simulink model "TestComputeProfileSource"  (R2025b)
settings: Solver=ode23t  StartTime=0.0  StopTime=15  MaxStep=1e-3  RelTol=1e-4
libraries: nesl_utility x5, fl_lib x1, datacenter_lib x1, simulink x1
settings Model: Creator=saprasad  LastModifiedBy=saprasad
settings SimscapeCC: SimscapeLogType=all  SimscapeLogName=simlog_TestComputeProfileSource  SimscapeLogLimitData=off

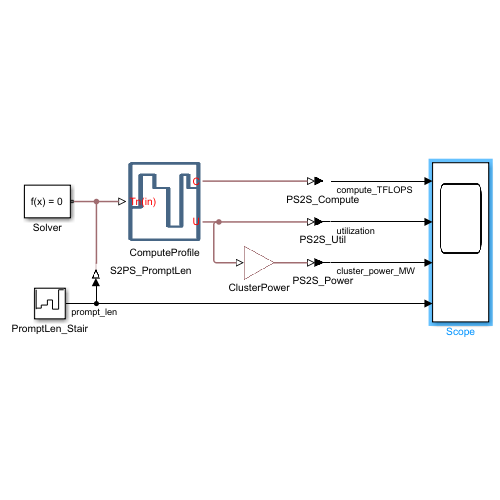
[thumbnail: Simulink's stored preview of the top-level diagram]
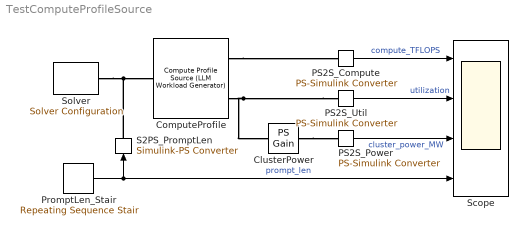
== system TestComputeProfileSource ==
  ClusterPower : fl_lib/Physical Signals/Functions/PS Gain  gain=1000 J/s
  ComputeProfile : datacenter_lib/Compute Profile Source (LLM Workload Generator)  gpuModel=GPUModel.B200  numGPUs=5184  workloadType=WorkloadType.Training  timeScale=10  tokenSource=TokenSource.External  showAdvanced=true  customPeakTFLOPS=1000  customHbmBW=4e12 1/s  hbmBW=8e12 1/s  interNodeBW=50e9 1/s  llmSize=LLMModelSize.GPT_175B  customNumParams_B=70  customNumLayers=80  customPrecision=2  parallelism=ParallelismStrategy.TP8_PP4  customTP=8  customPP=4  microBatch=8  globalBatch=12288  seqLength=2048  idleUtil=0.60  fwdUtil=0.92  bwdUtil=0.98  commSyncUtil=0.65  prompt_tokens=512  output_tokens=256  num_concurrent=8  batch_size=8  allreduce_latency=5e-6 s  baseInfUtil=0.08  baseInfFrac=0.10  MFU=0.85  checkpointOverhead=0.03  stragglerOverhead=0.02  trainableParamFrac=0.02  evalInterval=5  evalBatches=2  ft_checkpointOverhead=0.05  enableNoise=true  noiseAmplitude=0.05  stepJitter=0  enableFilter=false  filterTimeConstant=0.01 s  t_step_specify=off  t_step_priority=Low  t_step=0 s  t_step_nominal_specify=off  t_step_nominal_value=1  t_step_nominal_unit=s  phase_id_specify=off  phase_id_priority=None  phase_id=0  phase_id_nominal_specify=off  phase_id_nominal_value=1  phase_id_nominal_unit=1  utilization_specify=off  utilization_priority=None  utilization=0  utilization_nominal_specify=off  utilization_nominal_value=1  utilization_nominal_unit=1  step_count_specify=off  step_count_priority=None  step_count=0  step_count_nominal_specify=off  step_count_nominal_value=1  step_count_nominal_unit=1  tc_utilization_specify=off  tc_utilization_priority=None  tc_utilization=0  tc_utilization_nominal_specify=off  tc_utilization_nominal_value=1  tc_utilization_nominal_unit=1  hbm_utilization_specify=off  hbm_utilization_priority=None  hbm_utilization=0  hbm_utilization_nominal_specify=off  hbm_utilization_nominal_value=1  hbm_utilization_nominal_unit=1  tokens_per_sec_obs_specify=off  tokens_per_sec_obs_priority=None  tokens_per_sec_obs=0 1/s  tokens_per_sec_obs_nominal_specify=off  tokens_per_sec_obs_nominal_value=1  tokens_per_sec_obs_nominal_unit=1/s  ttft_obs_specify=off  ttft_obs_priority=None  ttft_obs=0 s  ttft_obs_nominal_specify=off  ttft_obs_nominal_value=1  ttft_obs_nominal_unit=s
      settings: InternalSimscapePortConfiguration="{\"Bottom\":[],\"Left\":[{\"id\":\"prompt_len_in\",\"label\":\"Tn(in)\",\"type\":\"input\"}],\"Right\":[{\"id\":\"compute\",\"label\":\"C\",\"type\":\"output\"},{\"id\":\"U\",\"label\":\"U\",\"type\":\"output\"}],\"Top\":[]}"
  PS2S_Compute : nesl_utility/PS-Simulink Converter  PhysicalDomain=network_engine_domain  SubClassName=ps_output  LeftPortType=input  RightPortType=output  PseudoPeriodic=off  Frequencies=[]  VectorFormat=inherit  Unit=1  AffineConversion=off
  PS2S_Power : nesl_utility/PS-Simulink Converter  PhysicalDomain=network_engine_domain  SubClassName=ps_output  LeftPortType=input  RightPortType=output  PseudoPeriodic=off  Frequencies=[]  VectorFormat=inherit  Unit=MW  AffineConversion=off
  PS2S_Util : nesl_utility/PS-Simulink Converter  PhysicalDomain=network_engine_domain  SubClassName=ps_output  LeftPortType=input  RightPortType=output  PseudoPeriodic=off  Frequencies=[]  VectorFormat=inherit  Unit=1  AffineConversion=off
  PromptLen_Stair : simulink/Sources/Repeating Sequence Stair  OutValues=[512 1024 2048 256 4096]  tsamp=1.5  OutMin=[]  OutMax=[]  OutDataTypeStr=double  OutputDataTypeScalingMode=double  OutDataType=fixdt(0,8)  ConRadixGroup=Best Precision: Vector-wise  OutScaling=2^-12
      settings: LibrarySourceBlock=|
      | hdlsllib/Sources/Repeating
      | Sequence
      | Stair
  S2PS_PromptLen : nesl_utility/Simulink-PS Converter  PhysicalDomain=network_engine_domain  SubClassName=ps_input  LeftPortType=input  RightPortType=output  PseudoPeriodic=off  Frequencies=[]  NoiseDistribution=none  NoiseParameters=[]  Unit=1  AffineConversion=off  FilteringAndDerivatives=provide  SimscapeFilterOrder=1  InputFilterTimeConstant=1e-3  UdotUserProvided=0
  Scope : Scope  NumInputPorts=4
      settings: ActiveDisplayYMinimum=6.0351148386603519E+6  ActiveDisplayYMaximum=1.2582629525104214E+7
  Solver : nesl_utility/Solver Configuration  PhysicalDomain=network_engine_domain  SubClassName=solver  LeftPortType=input  RightPortType=generic  Tones=[]  Harmonics=[]  SimulateNoise=off  Profile=off  UseLocalSampling=off  EnableSwitchedLinearOptims=on  FrequencyDomain=off  UseCCode=off  RelTol=0.001  AbsTol=0.001  MinStep=1e-09  ToWorkspace=off  RevertToSquareIcSolve=off  NumHomotopyIterations=100  PhasorMode=off  PhasorModeNumHarmonics=1  ConsistencySolver=NEWTON_XTOL_AFTER_FTOL  IndexReductionMethod=DerivativeReplacement  DoDC=off  ResidualTolerance=1e-09  ConsistencyTolSource=GLOBAL  ConsistencyAbsTol=0.001  ConsistencyRelTol=0.001  ConsistencyTolFactor=0.001  UseLocalSolver=off  LocalSolverChoice=NE_BACKWARD_EULER_ADVANCER  ResolveIndetEquations=on  FunctionEvalNumThread=1  LocalSolverSampleTime=0.001  DoFixedCost=off  MaxNonlinIter=3  MaxModeIter=2  ComputeImpulses=off  ImpulseIterations=2  LinearAlgebra=auto  LinearAlgebraNumThread=0  EquationFormulation=NE_TIME_EF  DelaysMemoryBudget=1024  AutomaticFiltering=on  FilteringTimeConstant=0.001  PartitionStorageMethod=AS_NEEDED  PartitionMemoryBudget=1024  PartitionMethod=ROBUST  MultibodyUseLocalSolver=off  MultibodyLocalSolverChoice=ODE1  MultibodyLocalSolverSampleTime=0.001
  wires:
  PromptLen_Stair/1 -> S2PS_PromptLen/1, Scope/4  "prompt_len"
  PS2S_Compute/1 -> Scope/1  "compute_TFLOPS"
  PS2S_Util/1 -> Scope/2  "utilization"
  PS2S_Power/1 -> Scope/3  "cluster_power_MW"
  connections:
  S2PS_PromptLen/RConn1 -- Solver/RConn1 -- ComputeProfile/LConn1
  ComputeProfile/RConn1 -- PS2S_Compute/LConn1
  PS2S_Util/LConn1 -- ClusterPower/LConn1 -- ComputeProfile/RConn2
  ClusterPower/RConn1 -- PS2S_Power/LConn1
